simulink model "GSSAM_sim"  (R2024b)
settings: Solver=VariableStepAuto  StartTime=0.0  StopTime=2  MaxStep=1e-2  RelTol=1e-3
InitFcn:
  | %% PWM
  | f = 20e3; % Hz
  | pwm_T = 1/f;
  | Ts = 1e-6;
  | 
  | %% Gerador
  | K_e = 5.4e-3; % Relação FEM/rotacao
  | p = 5; % Numero de pares de pólos
  | R_ger = 1.94; % mOhm - Conferir unidade no simulink
  | L_ger = 77; % uH - conferir unidade no simulink
  | 
  | %% Retificador trifásico
  | V_fwd = 1.46; % em Volts e I_fwd = 150A
  | R_on = (1.46-1.13)/(150 - 50); % Ohm - on resistance
  | G_off = 100/1200; % uS - off Conductance
  | 
  | %% Indutores e capacitores
  | C = 12000e-6; % F - Conferir unidade no simulink
  | 
  | %% Indutores
  | L = 80e-3; % H - Conferir unidade no simulink
  | R_ind = 0; %1e-6; % ohm - Conferir unidade no simulink
libraries: dspindex x1, cstblocks x1
settings Model: Creator=eric  LastModifiedBy=eric

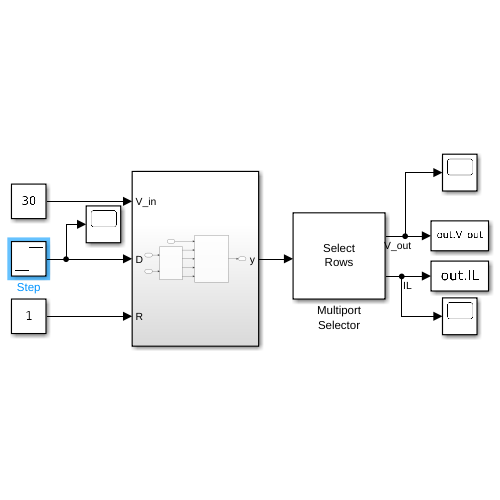
[thumbnail: Simulink's stored preview of the top-level diagram]
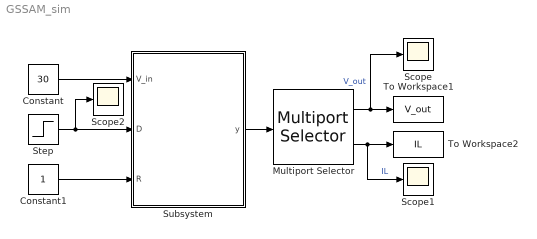
== system GSSAM_sim ==
  Constant : Constant  Value=30
  Constant1 : Constant
  Multiport Selector : dspindex/Multiport Selector  rowsOrCols=Rows  idxCellArray={ 4, [1:3]}  idxErrMode=Clip Index
      settings: LibrarySourceBlock=|
      | dsphdlsupportsigmgmt/Multiport
      | Selector
  Scope : Scope
  Scope1 : Scope
  Scope2 : Scope
  Step : Step  Before=0.25  After=0.3  SampleTime=0
  Subsystem : Subsystem
  To Workspace1 : ToWorkspace  VariableName=V_out  SampleTime=-1
  To Workspace2 : ToWorkspace  VariableName=IL  SampleTime=-1
      settings: Save2DSignal=2-D array (concatenate along first dimension)
  wires:
  Step/1 -> Scope2/1, Subsystem/2(D)
  Constant/1 -> Subsystem/1(V_in)
  Constant1/1 -> Subsystem/3(R)
  Subsystem/1(y) -> Multiport Selector/1
  Multiport Selector/1 -> Scope/1, To Workspace1/1  "V_out"
  Multiport Selector/2 -> Scope1/1, To Workspace2/1  "IL"

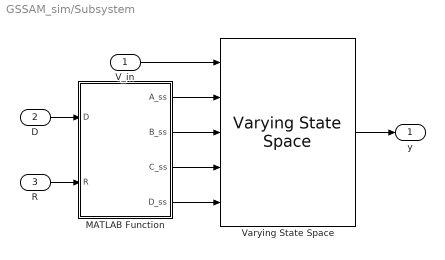
== system GSSAM_sim/Subsystem ==
  V_in : Inport
  D : Inport  Port=2
  R : Inport  Port=3
  MATLAB Function : MATLAB Function  TreatAsAtomicUnit=on
  Varying State Space : cstblocks/Linear Parameter Varying/Varying State Space  InitialConditionSource=internal  InitialCondition=0  xNames=''  OutputX=off  OutputDX=off  Feedthrough=on  InputX0=off  InputDX0=off  InputU0=off  InputY0=off
  y : Outport
  wires:
  R/1 -> MATLAB Function/2(R)
  MATLAB Function/4(D_ss) -> Varying State Space/5
  D/1 -> MATLAB Function/1(D)
  MATLAB Function/3(C_ss) -> Varying State Space/4
  MATLAB Function/2(B_ss) -> Varying State Space/3
  MATLAB Function/1(A_ss) -> Varying State Space/2
  V_in/1 -> Varying State Space/1
  Varying State Space/1 -> y/1

== matlab function GSSAM_sim/Subsystem/MATLAB Function ==
  data: A_ss output; B_ss output; C_ss output; D_ss output; D input; R input; C parameter; L parameter; R_ind parameter
function [A_ss, B_ss, C_ss, D_ss] = get_ss(D, R, C, L, R_ind)
    A_ss = function_A_0_order(C, D, L, R, R_ind);
    B_ss = function_B_0_order(L);
    C_ss = function_C_0_order();
    D_ss = zeros(4, 1);
end
